simulink model "sy3_08022311"  (R2022b)
settings: Solver=VariableStepAuto  StartTime=0.0  StopTime=50  RelTol=1e-3
settings Model: Creator=赵晨琨  LastModifiedBy=ASUS
settings SolverCC: AlgebraicLoopSolver=TrustRegion
settings DataIOCC: Refine=3
settings DebuggingCC: UnconnectedInputMsg=warning  UnconnectedOutputMsg=warning  UnconnectedLineMsg=warning  SFMachineParentedDataDiag=warning
settings ModelReferenceCC: EnableRefExpFcnMdlSchedulingChecks=on

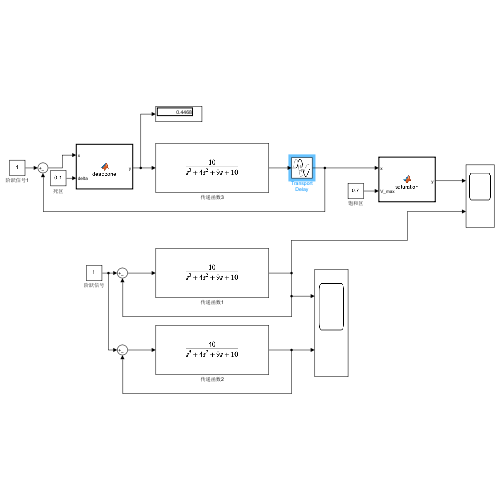
[thumbnail: Simulink's stored preview of the top-level diagram]
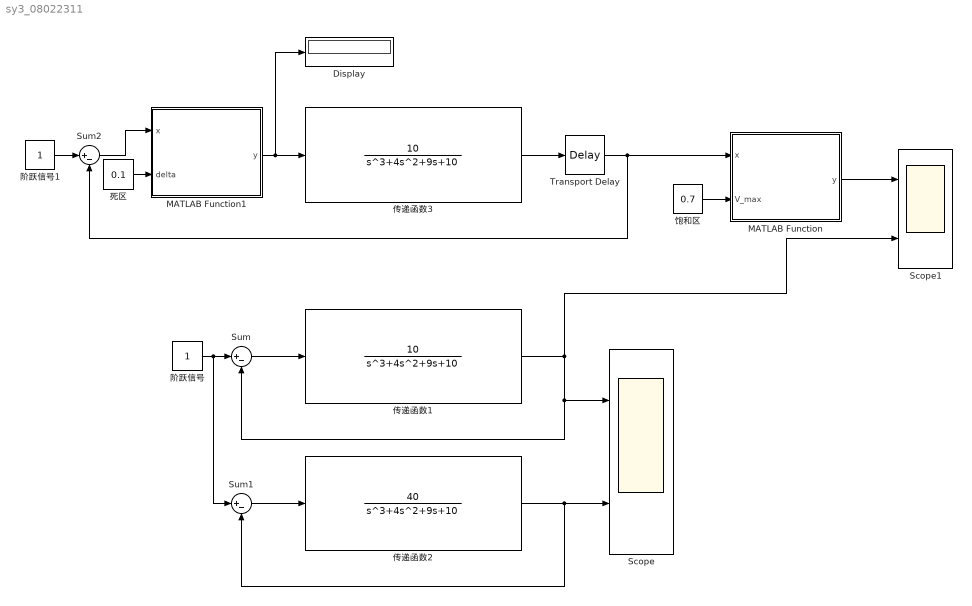
== system sy3_08022311 ==
  Display : Display
  MATLAB Function : MATLAB Function  TreatAsAtomicUnit=on
  MATLAB Function1 : MATLAB Function  TreatAsAtomicUnit=on
  Scope : Scope  NumInputPorts=2
  Scope1 : Scope  NumInputPorts=2
  Sum : Sum  Inputs=|+-
  Sum1 : Sum  Inputs=|+-
  Sum2 : Sum  Inputs=|+-
  Transport Delay : TransportDelay  DelayTime=0.5
  传递函数1 : TransferFcn  Numerator=[10]  Denominator=[1 4 9 10]
  传递函数2 : TransferFcn  Numerator=[40]  Denominator=[1 4 9 10]
  传递函数3 : TransferFcn  Numerator=[10]  Denominator=[1 4 9 10]
  死区 : Constant  Value=0.1
  阶跃信号 : Constant
  阶跃信号1 : Constant
  饱和区 : Constant  Value=0.7
  wires:
  Sum/1 -> 传递函数1/1
  传递函数1/1 -> Scope1/2, Scope/1, Sum/2
  传递函数2/1 -> Scope/2, Sum1/2
  Sum1/1 -> 传递函数2/1
  阶跃信号/1 -> Sum1/1, Sum/1
  阶跃信号1/1 -> Sum2/1
  MATLAB Function/1(y) -> Scope1/1
  饱和区/1 -> MATLAB Function/2(V_max)
  MATLAB Function1/1(y) -> Display/1, 传递函数3/1
  Sum2/1 -> MATLAB Function1/1(x)
  死区/1 -> MATLAB Function1/2(delta)
  传递函数3/1 -> Transport Delay/1
  Transport Delay/1 -> MATLAB Function/1(x), Sum2/2

== matlab function sy3_08022311/MATLAB Function ==
  data: x input; y output; V_max input
%饱和函数
function y = saturation(x, V_max)
    if x > V_max
        y = V_max;  % 上饱和
    elseif x < -V_max
        y = -V_max; % 下饱和
    else
        y = x;       % 非饱和区
    end
end

== matlab function sy3_08022311/MATLAB Function1 ==
  data: x input; y output; delta input
% 死区函数
function y = deadzone(x, delta)
    if abs(x) < delta
        y = 0;  % 输入信号在死区内时，输出为零
    else
        y = x - delta * sign(x);  % 输入信号在死区外时，输出为去掉死区的信号
    end
end
